simulink model "enginePropFixedwing"  (R2026a)
settings: configuration reference "standardSILConfiguraitonParams" (kept outside this file)
settings Model: Creator=Edison Altamirano  LastModifiedBy=Edison Altamirano
settings ConfigSetRef: SourceName=standardSILConfiguraitonParams  SourceLocation=Base Workspace

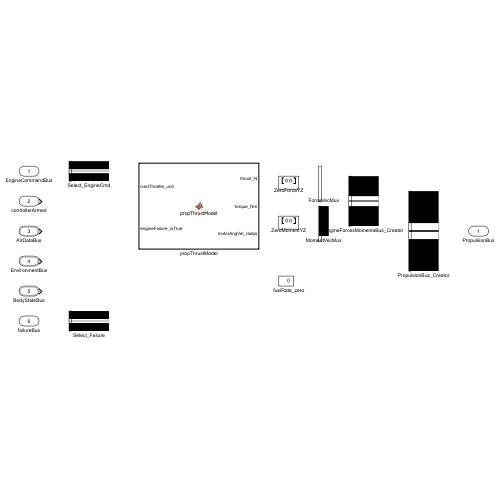
[thumbnail: Simulink's stored preview of the top-level diagram]
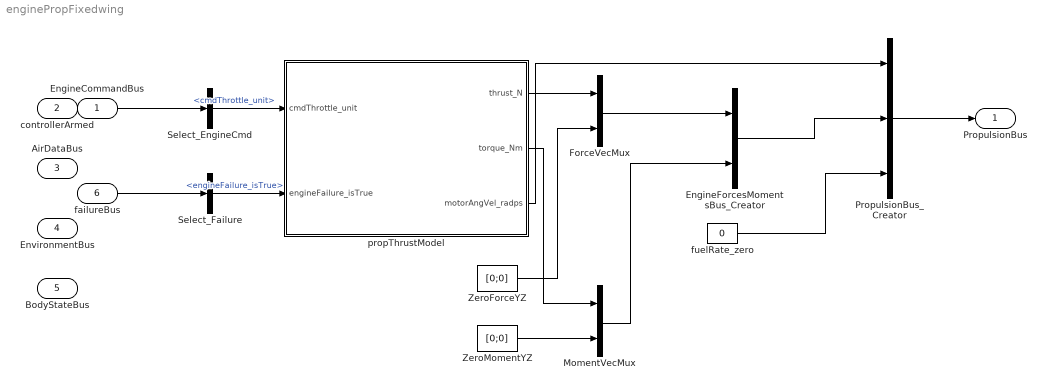
== system enginePropFixedwing ==
  EngineCommandBus : Inport  OutDataTypeStr=Bus: EngineCommandBus
  controllerArmed : Inport  Port=2
  AirDataBus : Inport  Port=3  OutDataTypeStr=Bus: AirDataBus
  EnvironmentBus : Inport  Port=4  OutDataTypeStr=Bus: EnvironmentBus
  BodyStateBus : Inport  Port=5  OutDataTypeStr=Bus: BodyStateBus
  failureBus : Inport  Port=6  OutDataTypeStr=Bus: FailureBus
  EngineForcesMomentsBus_Creator : BusCreator  Inputs=2  OutDataTypeStr=Bus: ComponentForcesMomentsBus
  ForceVecMux : Mux  Inputs=2
  MomentVecMux : Mux  Inputs=2
  PropulsionBus_Creator : BusCreator  Inputs=3  OutDataTypeStr=Bus: PropulsionBus
  Select_EngineCmd : BusSelector  OutputSignals=cmdThrottle_unit
  Select_Failure : BusSelector  OutputSignals=engineFailure_isTrue
  ZeroForceYZ : Constant  Value=[0;0]
  ZeroMomentYZ : Constant  Value=[0;0]
  fuelRate_zero : Constant  Value=0
  propThrustModel : MATLAB Function  TreatAsAtomicUnit=on
  PropulsionBus : Outport  OutDataTypeStr=Bus: PropulsionBus
  wires:
  EngineCommandBus/1 -> Select_EngineCmd/1
  fuelRate_zero/1 -> PropulsionBus_Creator/3
  failureBus/1 -> Select_Failure/1
  propThrustModel/1(thrust_N) -> ForceVecMux/1
  Select_Failure/1 -> propThrustModel/2(engineFailure_isTrue)  "<engineFailure_isTrue>"
  Select_EngineCmd/1 -> propThrustModel/1(cmdThrottle_unit)  "<cmdThrottle_unit>"
  propThrustModel/2(torque_Nm) -> MomentVecMux/1
  ZeroForceYZ/1 -> ForceVecMux/2
  PropulsionBus_Creator/1 -> PropulsionBus/1
  propThrustModel/3(motorAngVel_radps) -> PropulsionBus_Creator/1
  ZeroMomentYZ/1 -> MomentVecMux/2
  ForceVecMux/1 -> EngineForcesMomentsBus_Creator/1
  EngineForcesMomentsBus_Creator/1 -> PropulsionBus_Creator/2
  MomentVecMux/1 -> EngineForcesMomentsBus_Creator/2

== matlab function enginePropFixedwing/propThrustModel ==
  data: cmdThrottle_unit input; thrust_N output; engineFailure_isTrue input; torque_Nm output; motorAngVel_radps output
function [thrust_N, torque_Nm, motorAngVel_radps] = ...
    propThrustModel(cmdThrottle_unit, engineFailure_isTrue)
%#codegen
persistent motorAngVel_radps_state;
if isempty(motorAngVel_radps_state)
    motorAngVel_radps_state = 0;
end

% Single tractor propeller, electric motor -- see
% vehicle/common/setUpActuators.m 'fixedwing_plane' case for parameter
% sourcing. Constants inlined (not read from vehicleParams) per the same
% MATLAB-Function-block struct-compile constraint documented in
% optimAeroPX4SIL/CLAUDE.md section 3.
maxRPM = 9000;
maxAngVel_radps = maxRPM * 2 * pi / 60;
tauMotor_s = 0.15;
Ts_s = 0.01;
kct_nd = 3.6e-5;
kcp_nd = 2.24e-6;

if engineFailure_isTrue
    throttleCmd_nd = 0;
else
    throttleCmd_nd = max(min(cmdThrottle_unit, 1), 0);
end
targetAngVel_radps = throttleCmd_nd * maxAngVel_radps;

alpha = Ts_s / (tauMotor_s + Ts_s);
motorAngVel_radps_state = motorAngVel_radps_state + alpha * ...
    (targetAngVel_radps - motorAngVel_radps_state);

motorAngVel_radps = motorAngVel_radps_state;
thrust_N = kct_nd * motorAngVel_radps^2;
torque_Nm = -kcp_nd * motorAngVel_radps^2;
end
